simulink model "Natural_Sampling_EEE311L_Exp_04"  (R2025b)
settings: Solver=VariableStepAuto  StartTime=0.0  StopTime=10.0  RelTol=1e-3
libraries: dspfdesign x2
settings Model: Creator=fahim  LastModifiedBy=fahim

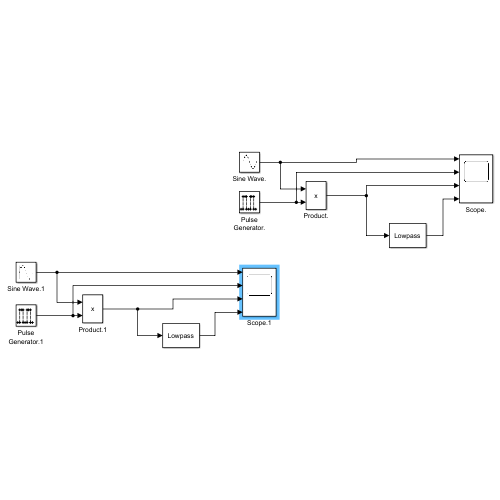
[thumbnail: Simulink's stored preview of the top-level diagram]
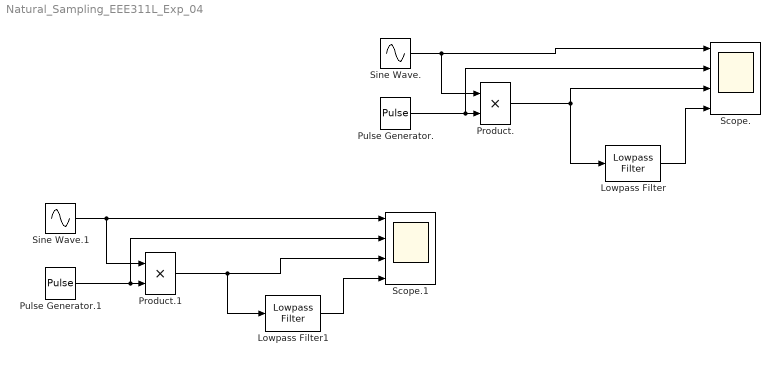
== system Natural_Sampling_EEE311L_Exp_04 ==
  Lowpass Filter : dspfdesign/Lowpass Filter  FilterType=IIR  DesignForMinimumOrder=on  FilterOrder=50  PassbandFrequency=200  StopbandFrequency=1000  PassbandRipple=0.1  StopbandAttenuation=80  SampleRateMode=Specify on dialog  SampleRate=44100  SimulateUsing=Interpreted execution  roundingMode=Floor  coeffsDataTypeStr=fixdt(1,16)
  Lowpass Filter1 : dspfdesign/Lowpass Filter  FilterType=IIR  DesignForMinimumOrder=on  FilterOrder=50  PassbandFrequency=30  StopbandFrequency=900  PassbandRipple=0.1  StopbandAttenuation=80  SampleRateMode=Specify on dialog  SampleRate=44100  SimulateUsing=Interpreted execution  roundingMode=Floor  coeffsDataTypeStr=fixdt(1,16)
  Product. : Product
  Product.1 : Product
  Pulse Generator. : DiscretePulseGenerator  Period=100  PulseWidth=50  SampleTime=0.001
  Pulse Generator.1 : DiscretePulseGenerator  Period=200  PulseWidth=100  SampleTime=0.001
  Scope. : Scope  NumInputPorts=4
      settings: ActiveDisplayString=3  Title=Sampled Message (Natural)  ActiveDisplayYMinimum=-1.2499753260701714  ActiveDisplayYMaximum=1.2499753260701714
  Scope.1 : Scope  NumInputPorts=4
      settings: ActiveDisplayString=4  Title=Reconstructed Signal  ActiveDisplayYMinimum=-0.62745906345523172  ActiveDisplayYMaximum=0.62211105923360066
  Sine Wave. : Sin  SineType=Sample based  Samples=1000  SampleTime=0.001
  Sine Wave.1 : Sin  SineType=Sample based  Samples=2000  SampleTime=0.001
  wires:
  Pulse Generator./1 -> Scope./2, Product./2
  Product./1 -> Lowpass Filter/1, Scope./3
  Sine Wave./1 -> Scope./1, Product./1
  Product.1/1 -> Lowpass Filter1/1, Scope.1/3
  Pulse Generator.1/1 -> Scope.1/2, Product.1/2
  Sine Wave.1/1 -> Scope.1/1, Product.1/1
  Lowpass Filter1/1 -> Scope.1/4
  Lowpass Filter/1 -> Scope./4
